simulink model "cannyHDL_2019b"  (R2019b)
settings: Solver=FixedStepDiscrete  StartTime=0.0  StopTime=totalPixels  RelTol=1e-3
values from neighbouring files (symbols this model uses):
  Gx_kernel = [-1 0 1 ... (first row only)    [canny.m]    (also in parameters.m)
  Gy_kernel = [1  2  1 ... (first row only)    [canny.m]    (also in parameters.m)
  kernel = [1  4  7  4 1 ... (first row only)    [parameters.m]
  maxVal = 100    [canny.m]    (also in parameters.m)
  minVal = 80    [canny.m]    (also in parameters.m)
libraries: visionhdlio x4, visionhdlfilter x3, visionhdlutilities x2, dsphdlmathfun x1, dspvision x1, simulink x1, hdlsllib x1
settings Model: SimulationMode=accelerator  Creator=lbai  LastModifiedBy=lbai
settings HardwareCC: ProdBitPerPointer=32  ProdBitPerSizeT=32  ProdBitPerPtrDiffT=32  ProdLargestAtomicFloat=None  ProdIntDivRoundTo=Undefined  ProdEndianess=Unspecified  ProdWordSize=32  ProdHWDeviceType=ASIC/FPGA->ASIC/FPGA  TargetBitPerPointer=64  TargetBitPerSizeT=64  TargetBitPerPtrDiffT=64  TargetLongLongMode=on  TargetIntDivRoundTo=Zero  TargetEndianess=LittleEndian  TargetWordSize=64  TargetHWDeviceType=Custom Processor->MATLAB Host Computer  ProdEqTarget=off

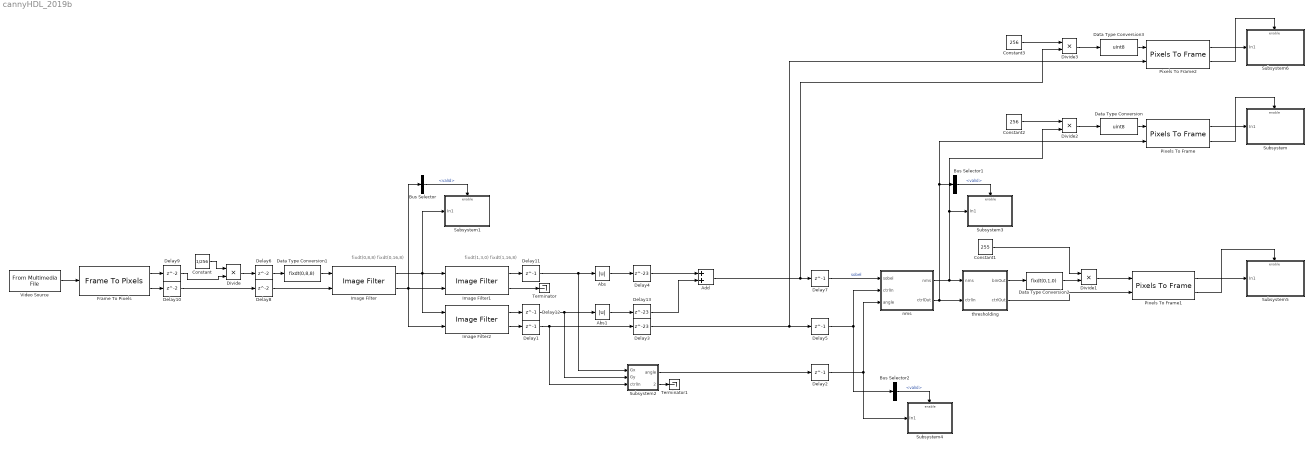
== system cannyHDL_2019b ==
  note: fixdt(1,3,0)
      | fixdt(1,16,8)
  note: fixdt(0,8,8)
      | fixdt(0,16,8)
  Abs : Abs
  Abs1 : Abs
  Add : Sum  OutDataTypeStr=Inherit: Same as accumulator  RndMeth=Ceiling
  Bus Selector : BusSelector  OutputSignals=valid
  Bus Selector1 : BusSelector  OutputSignals=valid
  Bus Selector2 : BusSelector  OutputSignals=valid
  Constant : Constant  Value=1/256  OutDataTypeStr=fixdt(0,16,16)  SampleTime=-1
  Constant1 : Constant  Value=255  OutDataTypeStr=uint8  SampleTime=-1
  Constant2 : Constant  Value=256  OutDataTypeStr=fixdt(0,16,0)  SampleTime=-1
  Constant3 : Constant  Value=256  OutDataTypeStr=fixdt(0,16,0)  SampleTime=-1
  Data Type Conversion : DataTypeConversion  OutDataTypeStr=uint8  SaturateOnIntegerOverflow=on
  Data Type Conversion1 : DataTypeConversion  OutDataTypeStr=fixdt(0,8,8)
  Data Type Conversion2 : DataTypeConversion  OutDataTypeStr=fixdt(0,1,0)
  Data Type Conversion3 : DataTypeConversion  OutDataTypeStr=uint8  SaturateOnIntegerOverflow=on
  Delay{1..2,5,7,11..12} (6 alike) : Delay  DelayLength=1
  Delay{6,8..10} (4 alike) : Delay
  Delay13 : Delay  DelayLength=23
  Delay3 : Delay  DelayLength=23
  Delay4 : Delay  DelayLength=23
  Divide{,1..3} (4 alike) : Product  Inputs=**
  Frame To Pixels : visionhdlio/Frame To Pixels  NumComponents=1  NumPixels=1  VideoFormat=240p  ActivePixelsPerLine=160  ActiveVideoLines=160  TotalPixelsPerLine=400  TotalVideoLines=400  StartingActiveLine=6  FrontPorch=120  SampleTime=0
      settings: SourceProductName=Vision HDL Toolbox  SourceProductBaseCode=VT
  Image Filter : visionhdlfilter/Image Filter  CoefficientsSource=Property  Coefficients=kernel  PaddingMethod=Constant  PaddingValue=0  LineBufferSize=2048  SimulateUsing=Code generation  roundingMode=Round  overflowMode=off  CoeffDataTypeStr=fixdt(0,8,8)  CoeffMin=[]  CoeffMax=[]  OutputDataTypeStr=fixdt(0,16,16)  OutputMin=[]  OutputMax=[]
      settings: SourceProductName=Vision HDL Toolbox  SourceProductBaseCode=VT
  Image Filter1 : visionhdlfilter/Image Filter  CoefficientsSource=Property  Coefficients=Gx_kernel  PaddingMethod=Constant  PaddingValue=0  LineBufferSize=2048  SimulateUsing=Code generation  roundingMode=Floor  overflowMode=off  CoeffDataTypeStr=fixdt(1,3,0)  CoeffMin=[]  CoeffMax=[]  OutputDataTypeStr=fixdt(1,16,13)  OutputMin=[]  OutputMax=[]
      settings: SourceProductName=Vision HDL Toolbox  SourceProductBaseCode=VT
  Image Filter2 : visionhdlfilter/Image Filter  CoefficientsSource=Property  Coefficients=Gy_kernel  PaddingMethod=Constant  PaddingValue=0  LineBufferSize=2048  SimulateUsing=Code generation  roundingMode=Floor  overflowMode=off  CoeffDataTypeStr=fixdt(1,3,0)  CoeffMin=[]  CoeffMax=[]  OutputDataTypeStr=fixdt(1,16,13)  OutputMin=[]  OutputMax=[]
      settings: SourceProductName=Vision HDL Toolbox  SourceProductBaseCode=VT
  Pixels To Frame : visionhdlio/Pixels To Frame  NumComponents=1  NumPixels=1  VideoFormat=240p  ActivePixelsPerLine=160  ActiveVideoLines=160  TotalPixelsPerLine=400  TotalVideoLines=400
      settings: SourceProductName=Vision HDL Toolbox  SourceProductBaseCode=VT
  Pixels To Frame1 : visionhdlio/Pixels To Frame  NumComponents=1  NumPixels=1  VideoFormat=240p  ActivePixelsPerLine=160  ActiveVideoLines=160  TotalPixelsPerLine=400  TotalVideoLines=400
      settings: SourceProductName=Vision HDL Toolbox  SourceProductBaseCode=VT
  Pixels To Frame2 : visionhdlio/Pixels To Frame  NumComponents=1  NumPixels=1  VideoFormat=240p  ActivePixelsPerLine=160  ActiveVideoLines=160  TotalPixelsPerLine=400  TotalVideoLines=400
      settings: SourceProductName=Vision HDL Toolbox  SourceProductBaseCode=VT
  Subsystem : Subsystem
  Subsystem1 : Subsystem
  Subsystem2 : Subsystem
  Subsystem3 : Subsystem
  Subsystem4 : Subsystem
  Subsystem5 : Subsystem
  Subsystem6 : Subsystem
  Terminator : Terminator
  Terminator1 : Terminator
  Video Source : dspvision/From Multimedia File  inputFilename=rhinos.avi  readRange=[1 Inf]  loop=on  numPlays=inf  outputStreams=Video only  videoDataType=uint8  audioDataType=int16  inheritSampleTime=off  userDefinedSampleTime=totalPixels  noAudioOutput=off  isIntensityVideo=off  fourcc=Intensity  colorVideoFormat=One multidimensional signal  outputEOF=off  dataOrg=Column-major  audioFrameSize=1024  computeAudioFrameSize=off  outSamplingMode=Sample based
      settings: SourceProductName=DSP System Toolbox  SourceProductBaseCode=DS
  nms : Subsystem
  thresholding : Subsystem
  wires:
  Video Source/1 -> Frame To Pixels/1
  Frame To Pixels/2 -> Delay10/1
  Image Filter/1 -> Subsystem1/1(In1), Image Filter2/1, Image Filter1/1
  Image Filter/2 -> Bus Selector/1, Image Filter2/2, Image Filter1/2
  Image Filter1/1 -> Delay11/1
  Image Filter2/1 -> Delay12/1
  Image Filter1/2 -> Terminator/1
  Abs/1 -> Delay4/1
  Divide1/1 -> Pixels To Frame1/1
  Abs1/1 -> Delay13/1
  Delay4/1 -> Add/1
  Delay7/1 -> nms/1(sobel)  "sobel"
  Subsystem2/1(angle) -> Delay2/1
  Delay1/1 -> Subsystem2/3(ctrlIn), Delay3/1
  Image Filter2/2 -> Delay1/1
  Constant/1 -> Divide/1
  Frame To Pixels/1 -> Delay9/1
  Delay6/1 -> Data Type Conversion1/1
  Delay8/1 -> Image Filter/2
  Delay10/1 -> Delay8/1
  Delay9/1 -> Divide/2
  Bus Selector/1 -> Subsystem1/Enable  "<valid>"
  Data Type Conversion1/1 -> Image Filter/1
  Delay11/1 -> Subsystem2/1(Gx), Abs/1
  Divide/1 -> Delay6/1
  Delay12/1 -> Subsystem2/2(Gy), Abs1/1
  Delay13/1 -> Add/2
  nms/2(ctrlOut) -> Pixels To Frame/2, Bus Selector1/1, thresholding/2(ctrlIn)
  thresholding/1(binOut) -> Data Type Conversion2/1
  Constant1/1 -> Divide1/1
  Data Type Conversion2/1 -> Divide1/2
  thresholding/2(ctrlOut) -> Pixels To Frame1/2
  Bus Selector1/1 -> Subsystem3/Enable  "<valid>"
  nms/1(nms) -> Divide2/2, Subsystem3/1(In1), thresholding/1(nms)
  Delay2/1 -> Subsystem4/1(In1), nms/3(angle)
  Bus Selector2/1 -> Subsystem4/Enable  "<valid>"
  Delay5/1 -> Bus Selector2/1, nms/2(ctrlIn)
  Pixels To Frame/1 -> Subsystem/1(In1)
  Pixels To Frame/2 -> Subsystem/Enable
  Data Type Conversion/1 -> Pixels To Frame/1
  Divide2/1 -> Data Type Conversion/1
  Constant2/1 -> Divide2/1
  Subsystem2/2(ctrlOut) -> Terminator1/1
  Pixels To Frame1/2 -> Subsystem5/Enable
  Pixels To Frame1/1 -> Subsystem5/1(In1)
  Constant3/1 -> Divide3/1
  Divide3/1 -> Data Type Conversion3/1
  Data Type Conversion3/1 -> Pixels To Frame2/1
  Pixels To Frame2/2 -> Subsystem6/Enable
  Pixels To Frame2/1 -> Subsystem6/1(In1)
  Add/1 -> Divide3/2, Delay7/1
  Delay3/1 -> Pixels To Frame2/2, Delay5/1

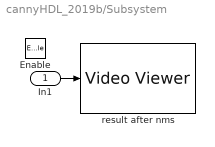
== system cannyHDL_2019b/Subsystem ==
  In1 : Inport
  Enable : EnablePort
  result after nms : VideoViewer  FigPos=[174 1057 876 790]
  wires:
  In1/1 -> result after nms/1

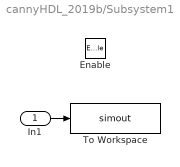
== system cannyHDL_2019b/Subsystem1 ==
  In1 : Inport
  Enable : EnablePort
  To Workspace : ToWorkspace  VariableName=simout  SaveFormat=Timeseries  SampleTime=-1
  wires:
  In1/1 -> To Workspace/1

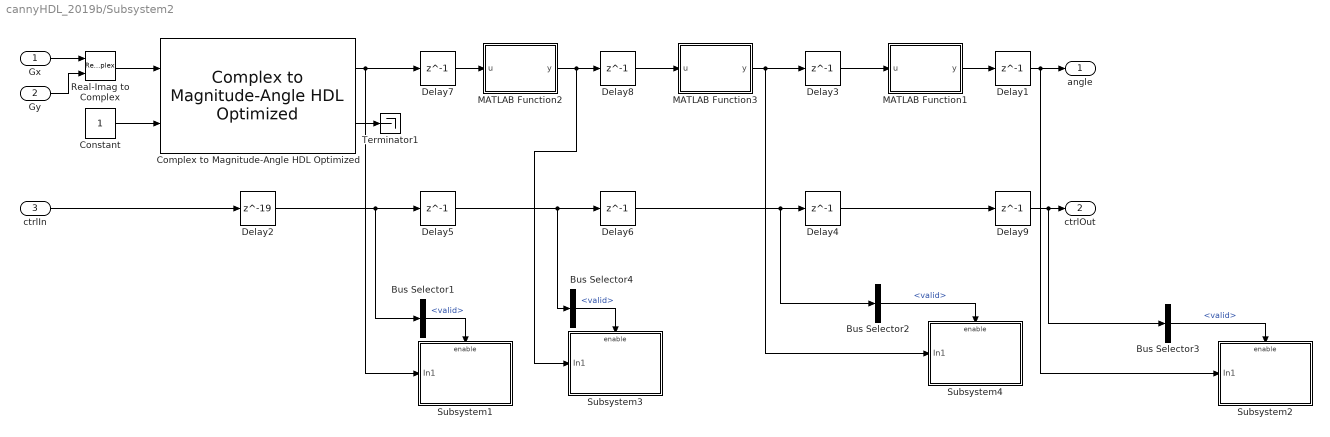
== system cannyHDL_2019b/Subsystem2 ==
  Gx : Inport
  Gy : Inport  Port=2
  ctrlIn : Inport  Port=3
  Bus Selector{1..4} (4 alike) : BusSelector  OutputSignals=valid
  Complex to Magnitude-Angle HDL Optimized : dsphdlmathfun/Complex to Magnitude-Angle HDL Optimized  NumIterationsSource=Auto  NumIterations=10  OutputFormat=Angle  AngleFormat=Normalized  ScaleOutput=on  SimulateUsing=Code generation
      settings: SourceProductName=DSP System Toolbox  SourceProductBaseCode=DS
  Constant : Constant  OutDataTypeStr=boolean  SampleTime=-1
  Delay{1,3..9} (8 alike) : Delay  DelayLength=1
  Delay2 : Delay  DelayLength=19
  MATLAB Function1 : MATLAB Function  TreatAsAtomicUnit=on
  MATLAB Function2 : MATLAB Function  TreatAsAtomicUnit=on
  MATLAB Function3 : MATLAB Function  TreatAsAtomicUnit=on
  Real-Imag to Complex : RealImagToComplex
  Subsystem1 : Subsystem
  Subsystem2 : Subsystem
  Subsystem3 : Subsystem
  Subsystem4 : Subsystem
  Terminator1 : Terminator
  angle : Outport
  ctrlOut : Outport  Port=2
  wires:
  Real-Imag to Complex/1 -> Complex to Magnitude-Angle HDL Optimized/1
  Constant/1 -> Complex to Magnitude-Angle HDL Optimized/2
  Complex to Magnitude-Angle HDL Optimized/2 -> Terminator1/1
  MATLAB Function1/1(y) -> Delay1/1
  ctrlIn/1 -> Delay2/1
  Bus Selector2/1 -> Subsystem4/Enable  "<valid>"
  Delay5/1 -> Bus Selector4/1, Delay6/1
  Gx/1 -> Real-Imag to Complex/1
  Gy/1 -> Real-Imag to Complex/2
  Delay6/1 -> Bus Selector2/1, Delay4/1
  Delay2/1 -> Bus Selector1/1, Delay5/1
  Bus Selector1/1 -> Subsystem1/Enable  "<valid>"
  Complex to Magnitude-Angle HDL Optimized/1 -> Delay7/1, Subsystem1/1(In1)
  MATLAB Function2/1(y) -> Subsystem3/1(In1), Delay8/1
  Delay7/1 -> MATLAB Function2/1(u)
  Delay8/1 -> MATLAB Function3/1(u)
  MATLAB Function3/1(y) -> Delay3/1, Subsystem4/1(In1)
  Delay3/1 -> MATLAB Function1/1(u)
  Delay4/1 -> Delay9/1
  Delay9/1 -> Bus Selector3/1, ctrlOut/1
  Delay1/1 -> Subsystem2/1(In1), angle/1
  Bus Selector3/1 -> Subsystem2/Enable  "<valid>"
  Bus Selector4/1 -> Subsystem3/Enable  "<valid>"

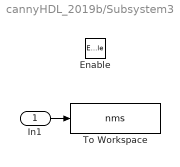
== system cannyHDL_2019b/Subsystem3 ==
  In1 : Inport
  Enable : EnablePort
  To Workspace : ToWorkspace  VariableName=nms  SaveFormat=Timeseries  SampleTime=-1
  wires:
  In1/1 -> To Workspace/1

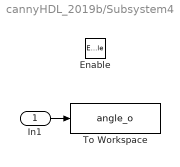
== system cannyHDL_2019b/Subsystem4 ==
  In1 : Inport
  Enable : EnablePort
  To Workspace : ToWorkspace  VariableName=angle_o  SaveFormat=Timeseries  SampleTime=-1
  wires:
  In1/1 -> To Workspace/1

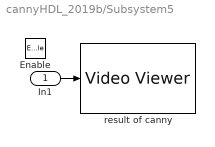
== system cannyHDL_2019b/Subsystem5 ==
  In1 : Inport
  Enable : EnablePort
  result of canny : VideoViewer  FigPos=[980 1004 886 820]
  wires:
  In1/1 -> result of canny/1

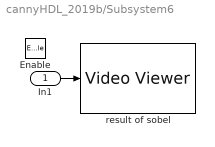
== system cannyHDL_2019b/Subsystem6 ==
  In1 : Inport
  Enable : EnablePort
  result of sobel : VideoViewer  FigPos=[174 1057 876 790]
  wires:
  In1/1 -> result of sobel/1

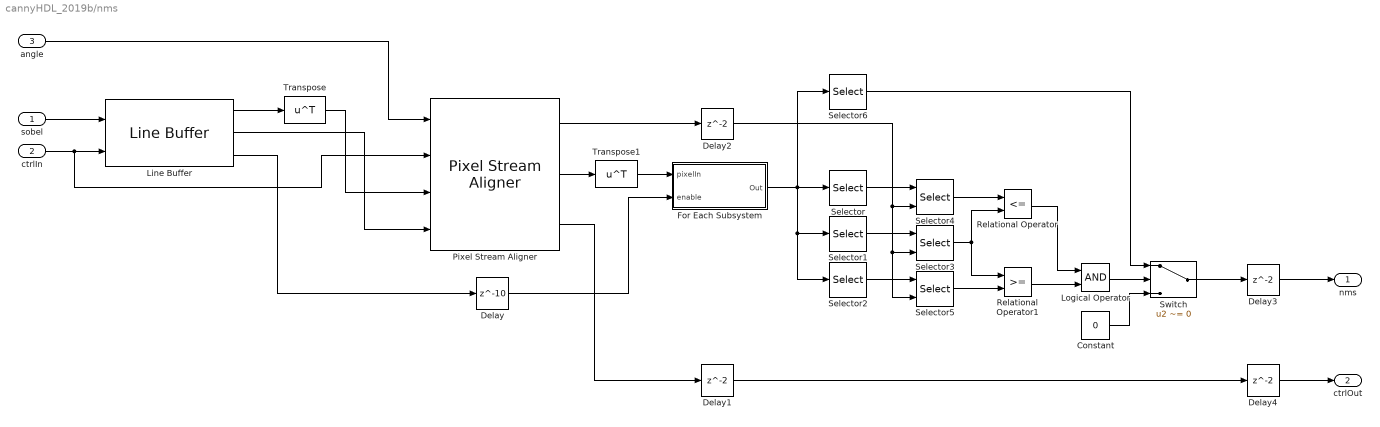
== system cannyHDL_2019b/nms ==
  sobel : Inport
  ctrlIn : Inport  Port=2
  angle : Inport  Port=3
  Constant : Constant  Value=0  OutDataTypeStr=fixdt(1,17,13)  SampleTime=-1
  Delay : Delay  DelayLength=10
  Delay{1..4} (4 alike) : Delay
  For Each Subsystem : Subsystem  TreatAsAtomicUnit=on
  Line Buffer : visionhdlutilities/Line Buffer  NeighborhoodSize=[3 3]  PaddingMethod=Constant  PaddingValue=0  LineBufferSize=2048*3  SimulateUsing=Code generation
      settings: SourceProductName=Vision HDL Toolbox  SourceProductBaseCode=VT
  Logical Operator : Logic  AllPortsSameDT=off  OutDataTypeStr=boolean
  Pixel Stream Aligner : visionhdlutilities/Pixel Stream Aligner  LineBufferSize=2048  MaximumNumberOfLines=10  SimulateUsing=Code generation
      settings: SourceProductName=Vision HDL Toolbox  SourceProductBaseCode=VT
  Relational Operator : RelationalOperator  Operator=<=  OutDataTypeStr=boolean  RndMeth=Simplest
  Relational Operator1 : RelationalOperator  OutDataTypeStr=boolean  RndMeth=Simplest
  Selector : Selector  InputPortWidth=9  IndexOptions=Index vector (dialog)  Indices=[2 1 4 3]  OutputSizes=1
  Selector1 : Selector  InputPortWidth=9  IndexOptions=Index vector (dialog)  Indices=[5 5 5 5]  OutputSizes=1
  Selector2 : Selector  InputPortWidth=9  IndexOptions=Index vector (dialog)  Indices=[8 9 6 7]  OutputSizes=1
  Selector3 : Selector  InputPortWidth=4  IndexOptions=Index vector (port)  Indices=[1 3]  OutputSizes=1
  Selector4 : Selector  InputPortWidth=4  IndexOptions=Index vector (port)  Indices=[1 3]  OutputSizes=1
  Selector5 : Selector  InputPortWidth=4  IndexOptions=Index vector (port)  Indices=[1 3]  OutputSizes=1
  Selector6 : Selector  InputPortWidth=9  IndexOptions=Index vector (dialog)  Indices=[5]  OutputSizes=1
  Switch : Switch  Criteria=u2 ~= 0
  Transpose : Math  Operator=transpose  RndMeth=Zero  SaturateOnIntegerOverflow=on
  Transpose1 : Math  Operator=transpose  RndMeth=Zero  SaturateOnIntegerOverflow=on
  nms : Outport
  ctrlOut : Outport  Port=2
  wires:
  Selector5/1 -> Relational Operator1/2
  Selector4/1 -> Relational Operator/1
  Constant/1 -> Switch/3
  For Each Subsystem/1(Out) -> Selector2/1, Selector1/1, Selector6/1, Selector/1
  sobel/1 -> Line Buffer/1
  Logical Operator/1 -> Switch/2
  Switch/1 -> Delay3/1
  Pixel Stream Aligner/1 -> Delay2/1
  ctrlIn/1 -> Pixel Stream Aligner/2, Line Buffer/2
  Selector3/1 -> Relational Operator/2, Relational Operator1/1
  Relational Operator1/1 -> Logical Operator/2
  Relational Operator/1 -> Logical Operator/1
  Selector/1 -> Selector4/1
  Selector1/1 -> Selector3/1
  Selector2/1 -> Selector5/1
  Line Buffer/2 -> Pixel Stream Aligner/4
  Line Buffer/1 -> Transpose/1
  Pixel Stream Aligner/2 -> Transpose1/1
  Line Buffer/3 -> Delay/1
  Delay/1 -> For Each Subsystem/2(enable)
  Transpose/1 -> Pixel Stream Aligner/3
  angle/1 -> Pixel Stream Aligner/1
  Pixel Stream Aligner/3 -> Delay1/1
  Transpose1/1 -> For Each Subsystem/1(pixelIn)
  Delay1/1 -> Delay4/1
  Selector6/1 -> Switch/1
  Delay2/1 -> Selector5/2, Selector3/2, Selector4/2
  Delay3/1 -> nms/1
  Delay4/1 -> ctrlOut/1

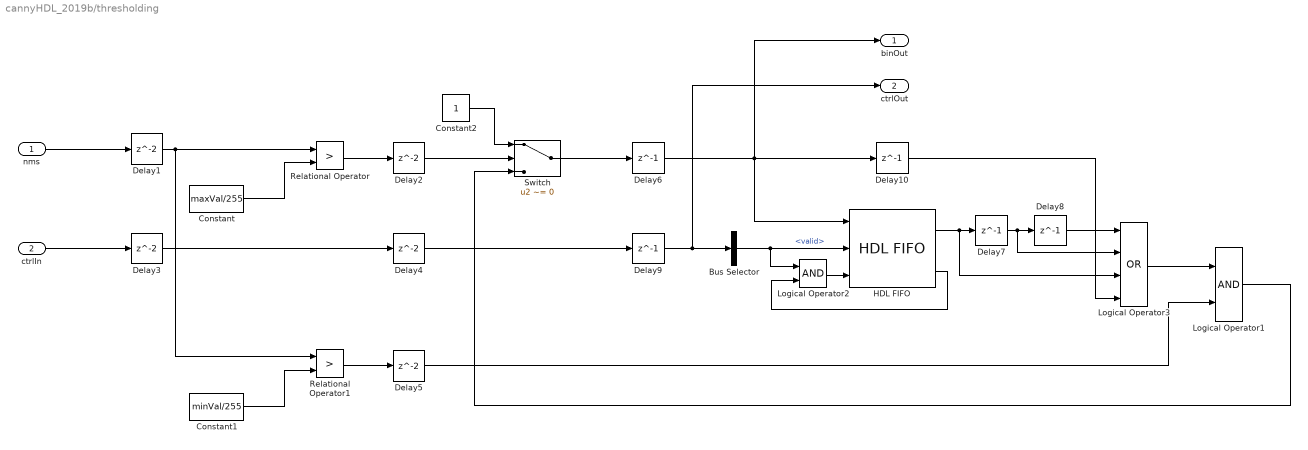
== system cannyHDL_2019b/thresholding ==
  nms : Inport
  ctrlIn : Inport  Port=2
  Bus Selector : BusSelector  OutputSignals=valid
  Constant : Constant  Value=maxVal/255  OutDataTypeStr=fixdt(0,16,16)  SampleTime=-1
  Constant1 : Constant  Value=minVal/255  OutDataTypeStr=fixdt(0,16,16)  SampleTime=-1
  Constant2 : Constant  OutDataTypeStr=boolean  SampleTime=-1
  Delay{1..5} (5 alike) : Delay
  Delay{6..10} (5 alike) : Delay  DelayLength=1
  HDL FIFO : hdlsllib/HDL RAMs/HDL FIFO  fifo_size=318  mode=Classic  ratio=1  push_msg=Warning  pop_msg=Warning  show_empty=off  show_full=on  show_num=off  LabelModeActiveChoice_Mode=Classic
      settings: SourceProductName=Simulink  SourceProductBaseCode=SL
  Logical Operator1 : Logic  AllPortsSameDT=off  OutDataTypeStr=boolean
  Logical Operator2 : Logic  AllPortsSameDT=off  OutDataTypeStr=boolean
  Logical Operator3 : Logic  Operator=OR  Inputs=4  AllPortsSameDT=off  OutDataTypeStr=boolean
  Relational Operator : RelationalOperator  Operator=>  OutDataTypeStr=boolean  RndMeth=Simplest
  Relational Operator1 : RelationalOperator  Operator=>  OutDataTypeStr=boolean  RndMeth=Simplest
  Switch : Switch  Criteria=u2 ~= 0
  binOut : Outport
  ctrlOut : Outport  Port=2
  wires:
  ctrlIn/1 -> Delay3/1
  nms/1 -> Delay1/1
  Delay1/1 -> Relational Operator/1, Relational Operator1/1
  Constant/1 -> Relational Operator/2
  Constant1/1 -> Relational Operator1/2
  Relational Operator1/1 -> Delay5/1
  Relational Operator/1 -> Delay2/1
  Delay3/1 -> Delay4/1
  Delay2/1 -> Switch/2
  Constant2/1 -> Switch/1
  Switch/1 -> Delay6/1
  Delay4/1 -> Delay9/1
  Logical Operator3/1 -> Logical Operator1/1
  Delay5/1 -> Logical Operator1/2
  Logical Operator1/1 -> Switch/3
  Delay7/1 -> Delay8/1, Logical Operator3/2
  HDL FIFO/2 -> Logical Operator2/2
  Delay6/1 -> binOut/1, Delay10/1, HDL FIFO/1
  Delay10/1 -> Logical Operator3/4
  Delay8/1 -> Logical Operator3/1
  Logical Operator2/1 -> HDL FIFO/3
  HDL FIFO/1 -> Delay7/1, Logical Operator3/3
  Bus Selector/1 -> Logical Operator2/1, HDL FIFO/2  "<valid>"
  Delay9/1 -> ctrlOut/1, Bus Selector/1

== system cannyHDL_2019b/Subsystem2/Subsystem1 ==
  In1 : Inport
  Enable : EnablePort
  To Workspace : ToWorkspace  VariableName=angle1  SaveFormat=Timeseries  SampleTime=-1
  wires:
  In1/1 -> To Workspace/1

== system cannyHDL_2019b/Subsystem2/Subsystem2 ==
  In1 : Inport
  Enable : EnablePort
  To Workspace : ToWorkspace  VariableName=angle4  SaveFormat=Timeseries  SampleTime=-1
  wires:
  In1/1 -> To Workspace/1

== system cannyHDL_2019b/Subsystem2/Subsystem3 ==
  In1 : Inport
  Enable : EnablePort
  To Workspace : ToWorkspace  VariableName=angle2  SaveFormat=Timeseries  SampleTime=-1
  wires:
  In1/1 -> To Workspace/1

== system cannyHDL_2019b/Subsystem2/Subsystem4 ==
  In1 : Inport
  Enable : EnablePort
  To Workspace : ToWorkspace  VariableName=angle3  SaveFormat=Timeseries  SampleTime=-1
  wires:
  In1/1 -> To Workspace/1

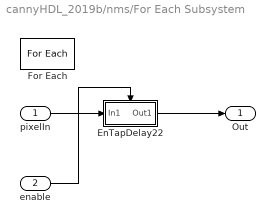
== system cannyHDL_2019b/nms/For Each Subsystem ==
  pixelIn : Inport  Partition=on  PartitionDimension=1  PartitionWidth=1  PartitionOffset=0
  enable : Inport  Port=2
  EnTapDelay22 : Subsystem
  For Each : ForEach  DisableCoverage=on
  Out : Outport  ConcatenationDimension=1  VectorParamsAs1DForOutWhenUnconnected=off
  wires:
  pixelIn/1 -> EnTapDelay22/1(In1)
  enable/1 -> EnTapDelay22/Enable
  EnTapDelay22/1(Out1) -> Out/1

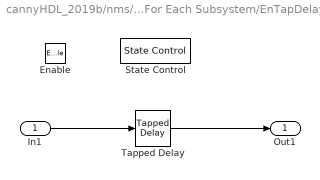
== system cannyHDL_2019b/nms/For Each Subsystem/EnTapDelay22 ==
  In1 : Inport
  Enable : EnablePort
  State Control : StateControl  StateControl=Synchronous
  Tapped Delay : simulink/Discrete/Tapped Delay  vinit=0.0  samptime=-1  NumDelays=3  DelayOrder=Oldest  includeCurrent=off
  Out1 : Outport  VectorParamsAs1DForOutWhenUnconnected=off
  wires:
  In1/1 -> Tapped Delay/1
  Tapped Delay/1 -> Out1/1

== matlab function cannyHDL_2019b/Subsystem2/MATLAB Function1 ==
  data: u input; y output
function y = fcn(u)

    u_temp = u-0.125;
    if u_temp<=0
        y = uint8(0);
    elseif u_temp<=0.25
        y = uint8(1);
    elseif u_temp<=0.5
        y = uint8(2);
    elseif u_temp<=0.75
        y = uint8(3);
    else
        y = uint8(0);
    end

== matlab function cannyHDL_2019b/Subsystem2/MATLAB Function2 ==
  data: u input; y output
function y = fcn(u)

    if u<=-0.5
        y = u+1;
    elseif u>0.5
        y = u-1;
    else
        y = fi(u,1,20,18);
    end

== matlab function cannyHDL_2019b/Subsystem2/MATLAB Function3 ==
  data: u input; y output
function y = fcn(u)
    
    if u<0
        y = abs(u-0.5);
    else
        y = fi(u,1,21,18);
    end
